simulink model "FixedwingPlaneAeroCoefficientsModel"  (R2026a)
settings: configuration reference "standardSILConfiguraitonParams" (kept outside this file)
settings Model: Creator=Edison Altamirano  LastModifiedBy=Edison Altamirano
settings ConfigSetRef: SourceName=standardSILConfiguraitonParams  SourceLocation=Base Workspace

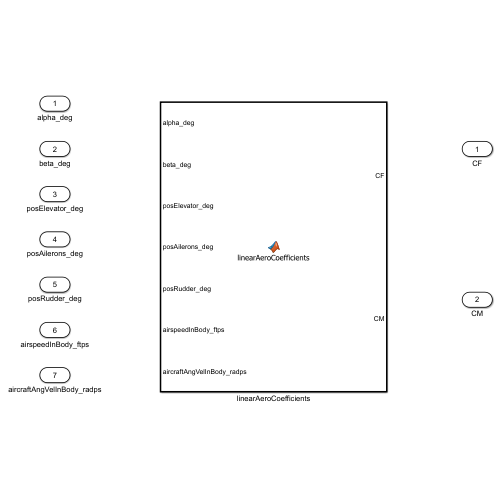
[thumbnail: Simulink's stored preview of the top-level diagram]
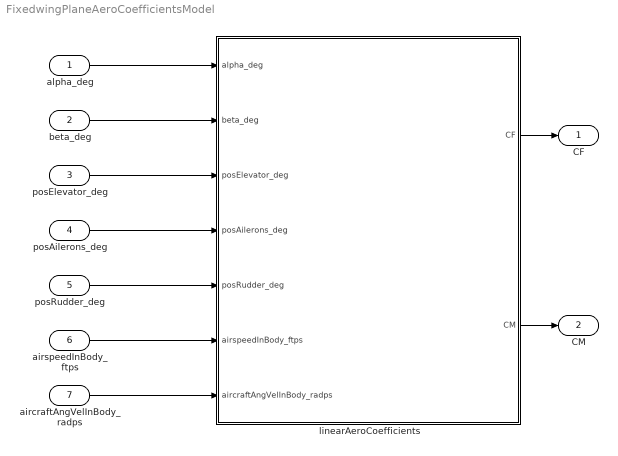
== system FixedwingPlaneAeroCoefficientsModel ==
  alpha_deg : Inport
  beta_deg : Inport  Port=2
  posElevator_deg : Inport  Port=3
  posAilerons_deg : Inport  Port=4
  posRudder_deg : Inport  Port=5
  airspeedInBody_ftps : Inport  Port=6  PortDimensions=3
  aircraftAngVelInBody_radps : Inport  Port=7  PortDimensions=3
  linearAeroCoefficients : MATLAB Function  TreatAsAtomicUnit=on
  CF : Outport
  CM : Outport  Port=2
  wires:
  linearAeroCoefficients/1(CF) -> CF/1
  airspeedInBody_ftps/1 -> linearAeroCoefficients/6(airspeedInBody_ftps)
  alpha_deg/1 -> linearAeroCoefficients/1(alpha_deg)
  beta_deg/1 -> linearAeroCoefficients/2(beta_deg)
  posRudder_deg/1 -> linearAeroCoefficients/5(posRudder_deg)
  posElevator_deg/1 -> linearAeroCoefficients/3(posElevator_deg)
  posAilerons_deg/1 -> linearAeroCoefficients/4(posAilerons_deg)
  aircraftAngVelInBody_radps/1 -> linearAeroCoefficients/7(aircraftAngVelInBody_radps)
  linearAeroCoefficients/2(CM) -> CM/1

== matlab function FixedwingPlaneAeroCoefficientsModel/linearAeroCoefficients ==
  data: alpha_deg input; CF output; beta_deg input; posElevator_deg input; posAilerons_deg input; posRudder_deg input; airspeedInBody_ftps input; aircraftAngVelInBody_radps input; CM output
function [CF, CM] = linearAeroCoefficients(alpha_deg, beta_deg, posElevator_deg, posAilerons_deg, posRudder_deg, airspeedInBody_ftps, aircraftAngVelInBody_radps)
%#codegen
% Linear stability-derivative aero model for a light (Funray-class) ala-fija
% RC/GA airframe. See build_FixedwingPlaneAeroCoefficientsModel.m header and
% PLAN_VEHICULOS_AEREOS_Y_MARINOS_SITL.md for sourcing/derivation of every
% constant below. All constants inlined as local values (not read from a
% struct-returning params function) -- MATLAB Function blocks in this MATLAB
% release fail to compile a call to a large-nested-struct-returning function,
% see optimAeroPX4SIL/CLAUDE.md section 3.

% Funray-derived reference geometry
bRef_m = 2.0;
cRef_m = 0.1853;

% Longitudinal linear stability/control derivatives (per rad)
CL0 = 0.05; CLalpha = 5.16; CLde = 0.5; CLq = 7.0;
CD0 = 0.035; kInducedDrag = 0.0347;
Cm0 = 0.02; Cmalpha = -1.0; Cmde = -1.5; Cmq = -15.0;

% Lateral-directional linear stability/control derivatives (per rad)
CYbeta = -0.5; CYdr = 0.15; CYp = -0.05; CYr = 0.2;
Clbeta = -0.03; Clda = 0.15; Cldr = 0.01; Clp = -0.5; Clr = 0.1;
Cnbeta = 0.08; Cnda = -0.01; Cndr = -0.08; Cnp = -0.02; Cnr = -0.15;

alpha_rad = deg2rad(alpha_deg);
beta_rad = deg2rad(beta_deg);
elevator_rad = deg2rad(posElevator_deg);
aileron_rad = deg2rad(posAilerons_deg);
rudder_rad = deg2rad(posRudder_deg);

V_mps = norm(airspeedInBody_ftps) * 0.3048;
VforRates_mps = max(V_mps, 1.0);
pRate_radps = aircraftAngVelInBody_radps(1);
qRate_radps = aircraftAngVelInBody_radps(2);
rRate_radps = aircraftAngVelInBody_radps(3);
pHat = pRate_radps * bRef_m / (2 * VforRates_mps);
qHat = qRate_radps * cRef_m / (2 * VforRates_mps);
rHat = rRate_radps * bRef_m / (2 * VforRates_mps);

CL = CL0 + CLalpha * alpha_rad + CLde * elevator_rad + CLq * qHat;
CD = CD0 + kInducedDrag * CL^2;
CY = CYbeta * beta_rad + CYdr * rudder_rad + CYp * pHat + CYr * rHat;

rollMomentCoefficient_nd = Clbeta * beta_rad + Clda * aileron_rad + ...
    Cldr * rudder_rad + Clp * pHat + Clr * rHat;
pitchMomentCoefficient_nd = Cm0 + Cmalpha * alpha_rad + Cmde * elevator_rad + Cmq * qHat;
yawMomentCoefficient_nd = Cnbeta * beta_rad + Cnda * aileron_rad + ...
    Cndr * rudder_rad + Cnp * pHat + Cnr * rHat;

% Wind-axes (CL,CD) -> body-axes (CX,CZ); CY needs no rotation at this
% linearized fidelity level (small-beta approximation).
CXTotal = -CD * cos(alpha_rad) + CL * sin(alpha_rad);
CZTotal = -CD * sin(alpha_rad) - CL * cos(alpha_rad);

CF = [CXTotal; CY; CZTotal];
CM = [rollMomentCoefficient_nd; pitchMomentCoefficient_nd; yawMomentCoefficient_nd];
end
